simulink model "InterfazOriginalv1Simu2016a"  (R2016a)
settings: Solver=FixedStepAuto  StartTime=10  StopTime=150  FixedStep=0.001  RelTol=1e-3
model workspace (MAT data in the model file):
  g_density = 5
libraries: simulink_extras x9, dspnetwork x7, etargetslib x5, dspfdesign x1
settings Model: Creator=Flight Test Lab  LastModifiedBy=Manolo
settings SolverCC: AutoInsertRateTranBlk=on
settings DataIOCC: SaveFormat=StructureWithTime
settings OptimizationCC: BlockReduction=off  DefaultUnderspecifiedDataType=single  OptimizeBlockIOStorage=off  BufferReuse=off  GlobalBufferReuse=off  ExpressionFolding=off  LocalBlockOutputs=off
settings DebuggingCC: SFUnexpectedBacktrackingDiag=error  SFNoUnconditionalDefaultTransitionDiag=error
settings HardwareCC: ProdWordSize=32  ProdHWDeviceType=Specified
settings RTWCC: Description=Generic Real-Time Target  TargetLang=C++  RTWCompilerOptimization=on
settings CodeAppCC: MaxIdLength=95
settings GRTTargetCC: TargetLangStandard=C++03 (ISO)  GeneratePreprocessorConditionals=Use local settings  MultiInstanceERTCode=on  CodeInterfacePackaging=C++ class
settings ConfigComp: CovMetricSettings=dwe  CovHtmlReporting=off  CovSaveCumulativeToWorkspaceVar=off  CovSaveSingleToWorkspaceVar=off  CovExternalEMLEnable=on

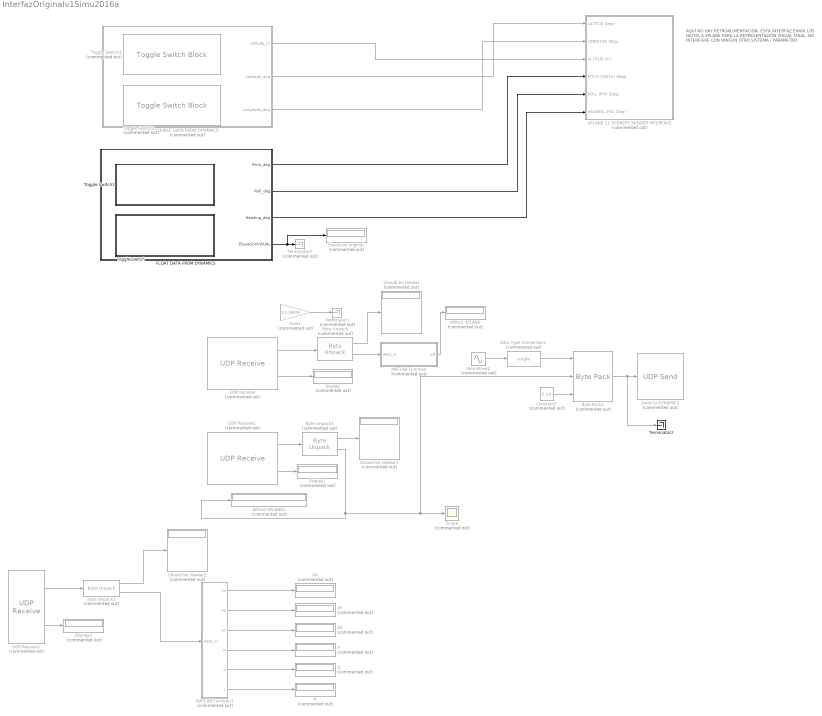
== system InterfazOriginalv1Simu2016a ==
  note: AQUÍ NO HAY RETROALIMENTACIÓN. ESTA INTERFAZ ENVÍA LOS DATOS
      | A XPLANE PARA LA REPRESENTACIÓN VISUAL FINAL, NO INTERFIERE CON
      | NINGUN OTRO SISTEMA / PARÁMETRO
  " DOUBLE DATA FROM DYNAMICS" : Subsystem  Commented=on
  " FLOAT DATA FROM DYNAMICS" : Subsystem
  " XPLANE 11 SCENERY RENDER INTERFACE" : Subsystem  Commented=on
  AX : Display  Commented=on
  AY : Display  Commented=on
  AZ : Display  Commented=on
  Altitud XPLANE : Display  Commented=on
  Altitud XPLANE2 : Display  Commented=on
      settings: Decimation=5
  Byte Pack1 : etargetslib/Byte Pack  Commented=on  datatypes={'single','single','single'}  byteAlign=1
  Byte Unpack : etargetslib/Byte Unpack  Commented=on  dimensions={5,[1,9]}  datatypes={'uint8','single'}  byteAlign=1
  Byte Unpack1 : etargetslib/Byte Unpack  Commented=on  dimensions={5,1}  datatypes={'uint8','single'}  byteAlign=1
  Byte Unpack3 : etargetslib/Byte Unpack  Commented=on  dimensions={5,[9,8]}  datatypes={'uint8','single'}  byteAlign=1
  Constant7 : Constant  Commented=on  Value=5.14  OutDataTypeStr=single
  Data Type Conversion1 : DataTypeConversion  Commented=on  OutDataTypeStr=single
  Display : Display  Commented=on
  Display1 : Display  Commented=on
  Display3 : Display  Commented=on
  Elevacion original : Display  Commented=on
      settings: Decimation=5
  Gain1 : Gain  Commented=on  Gain=1/3.28084
  MATLAB Function : MATLAB Function  Commented=on  TreatAsAtomicUnit=on
  MATLAB Function1 : MATLAB Function  Commented=on  TreatAsAtomicUnit=on
  P : Display  Commented=on
  Q : Display  Commented=on
  R : Display  Commented=on
  Scope : Scope  Commented=on
  Send to DYNAMICS : dspnetwork/UDP Send  Commented=on  remoteURL='1.1.1.1'  remotePort=19750  localURL='0.0.0.0'  localPortSource=Automatically determine  localPort=19750  sampletime=-1  blockPlatform=[]  separateLengthPort=0
  Should be Header : Display  Commented=on
  Should be Header1 : Display  Commented=on
  Should be Header2 : Display  Commented=on
  Sine Wave1 : Sin  Commented=on  Amplitude=90  SampleTime=0
  Terminator1 : Terminator  Commented=on
  Terminator2 : Terminator
  Terminator3 : Terminator  Commented=on
  Toggle Switch : Subsystem  DialogController=hmiCreateDDGDialog  IsWebBlock=on  mask(MWDashboardBlock){webBlockId=9a99a978-ce7c-43f5-ad35-1dbae24a8aa3, webBlockType=toggleswitch, ShowInLibBrowser=on, ShowInitialText=on, HMISrcModelName=InterfazOriginalv1Simu2016a}
      mask prompts: webBlockId "WebBlock Id"; webBlockType "WebBlock Type"; HMISrcModelName "Source Model"
      mask help: Set on/off value to tune parameters or variables.
      mask Help: helpview([docroot '/mapfiles/simulink.map'], 'hmi_switch')
      mask Display:
      | if strcmp(get_param(bdroot(gcb),'BlockDiagramType'),'library')
      |  image([(matlabroot) '/toolbox/simulink/hmi/icons/ToggleSwitch.png'])
      | end
  Toggle Switch1 : Subsystem  DialogController=hmiCreateDDGDialog  IsWebBlock=on  mask(MWDashboardBlock){webBlockId=7adb6560-95fd-42cd-ad0e-2d161efe3a99, webBlockType=toggleswitch, ShowInLibBrowser=on, ShowInitialText=on, HMISrcModelName=InterfazOriginalv1Simu2016a}
      mask prompts: webBlockId "WebBlock Id"; webBlockType "WebBlock Type"; HMISrcModelName "Source Model"
      mask help: Set on/off value to tune parameters or variables.
      mask Help: helpview([docroot '/mapfiles/simulink.map'], 'hmi_switch')
      mask Display:
      | if strcmp(get_param(bdroot(gcb),'BlockDiagramType'),'library')
      |  image([(matlabroot) '/toolbox/simulink/hmi/icons/ToggleSwitch.png'])
      | end
  Toggle Switch2 : ToggleSwitchBlock  Commented=on  WebBlockId=552  LabelPosition=Hide
      settings: Values={{'Replay Archivo', 'Conexión En Tiempo Real'}, [-1 1]}
  Toggle Switch3 : ToggleSwitchBlock  Commented=on  WebBlockId=553  LabelPosition=Hide
      settings: Values={{'No grabar', 'Grabar datos'}, [-1 1]}
  UDP Receive : dspnetwork/UDP Receive  Commented=on  localURL='0.0.0.0'  localPort=49004  remoteURL='127.0.0.1'  remotePort=-1  recvBufferSize=8192  dims=41  signalDatatype=uint8  isVarSize=off  showBlockingTime=off  blockingTime=0  sampletime=inf  blockPlatform=[]
  UDP Receive1 : dspnetwork/UDP Receive  Commented=on  localURL='0.0.0.0'  localPort=49010  remoteURL='127.0.0.1'  remotePort=-1  recvBufferSize=8192  dims=9  signalDatatype=uint8  isVarSize=off  showBlockingTime=off  blockingTime=0  sampletime=inf  blockPlatform=[]
  UDP Receive3 : dspnetwork/UDP Receive  Commented=on  localURL='0.0.0.0'  localPort=49004  remoteURL='127.0.0.1'  remotePort=-1  recvBufferSize=8192  dims=293  signalDatatype=uint8  isVarSize=off  showBlockingTime=off  blockingTime=0  sampletime=inf  blockPlatform=[]
  wires:
  Sine Wave1/1 -> Data Type Conversion1/1
  Constant7/1 -> Byte Pack1/3
  Byte Pack1/1 -> Terminator2/1, Send to DYNAMICS/1
  Data Type Conversion1/1 -> Byte Pack1/1
  UDP Receive/2 -> Display/1
  Byte Unpack/1 -> Should be Header/1
  UDP Receive/1 -> Byte Unpack/1
  Byte Unpack/2 -> MATLAB Function/1(data_in)
  MATLAB Function/1(alt) -> Altitud XPLANE/1
  " DOUBLE DATA FROM DYNAMICS"/2(Latitude_deg) -> " XPLANE 11 SCENERY RENDER INTERFACE"/1(LATITUD (Deg))
  " DOUBLE DATA FROM DYNAMICS"/3(Longitude_deg) -> " XPLANE 11 SCENERY RENDER INTERFACE"/2(LONGITUD (Deg))
  " FLOAT DATA FROM DYNAMICS"/1(Pitch_deg) -> " XPLANE 11 SCENERY RENDER INTERFACE"/4(PITCH (THETA) (Deg))
  " FLOAT DATA FROM DYNAMICS"/2(Roll_deg) -> " XPLANE 11 SCENERY RENDER INTERFACE"/5(ROLL (PHI) (Deg))
  " FLOAT DATA FROM DYNAMICS"/3(Heading_deg) -> " XPLANE 11 SCENERY RENDER INTERFACE"/6(HEADING (PSI) (Deg))
  " DOUBLE DATA FROM DYNAMICS"/1("altitude_m ") -> " XPLANE 11 SCENERY RENDER INTERFACE"/3(ALTITUD (m))
  UDP Receive1/2 -> Display1/1
  UDP Receive1/1 -> Byte Unpack1/1
  Byte Unpack1/1 -> Should be Header1/1
  Byte Unpack1/2 -> Byte Pack1/2, Scope/1, Altitud XPLANE2/1
  " FLOAT DATA FROM DYNAMICS"/4("ElevacionVISUAL ") -> Elevacion original/1, Terminator3/1
  Gain1/1 -> Terminator1/1
  MATLAB Function1/4(p) -> P/1
  MATLAB Function1/6(r) -> R/1
  MATLAB Function1/5(q) -> Q/1
  MATLAB Function1/2(ay) -> AY/1
  MATLAB Function1/3(az) -> AZ/1
  MATLAB Function1/1(ax) -> AX/1
  Byte Unpack3/1 -> Should be Header2/1
  Byte Unpack3/2 -> MATLAB Function1/1(data_in)
  UDP Receive3/1 -> Byte Unpack3/1
  UDP Receive3/2 -> Display3/1

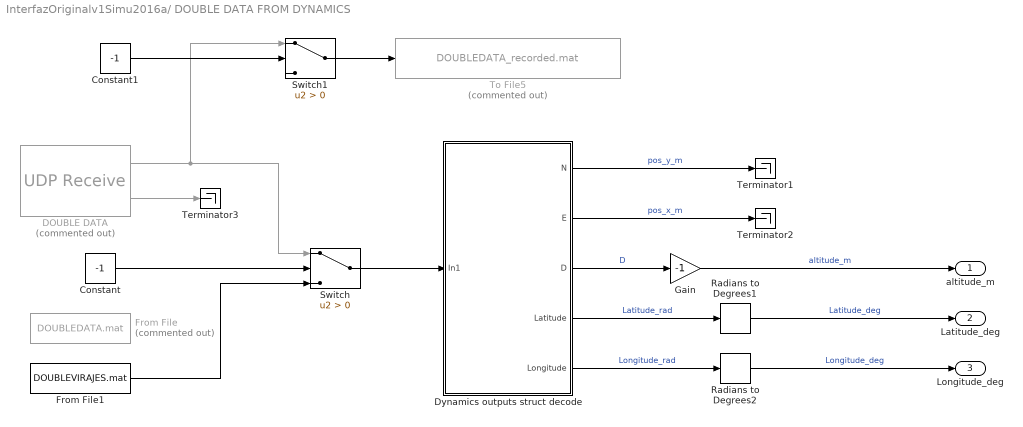
== system InterfazOriginalv1Simu2016a/ DOUBLE DATA FROM DYNAMICS ==
  Constant : Constant  Value=-1
  Constant1 : Constant  Value=-1
  DOUBLE DATA : dspnetwork/UDP Receive  Commented=on  localURL='0.0.0.0'  localPort=19700  remoteURL='0.0.0.0'  remotePort=-1  recvBufferSize=300  dims=5  signalDatatype=double  isVarSize=off  showBlockingTime=on  blockingTime=0  sampletime=0.001  blockPlatform=WINDOWS
  Dynamics outputs struct decode : Subsystem
  From File : FromFile  Commented=on  FileName=DOUBLEDATA.mat
  From File1 : FromFile  FileName=DOUBLEVIRAJES.mat
  Gain : Gain  Gain=-1
  Radians to Degrees1 : simulink_extras/Transformations/Radians to Degrees
  Radians to Degrees2 : simulink_extras/Transformations/Radians to Degrees
  Switch : Switch  Criteria=u2 > Threshold
  Switch1 : Switch  Criteria=u2 > Threshold
  Terminator1 : Terminator
  Terminator2 : Terminator
  Terminator3 : Terminator
  To File5 : ToFile  Commented=on  Filename=DOUBLEDATA_recorded.mat  MatrixName=DOUBLEDATA_recorded  SaveFormat=Timeseries  SampleTime=0.001
      settings: Decimation=16
  "altitude_m " : Outport
  Latitude_deg : Outport  Port=2
  Longitude_deg : Outport  Port=3
  wires:
  Dynamics outputs struct decode/3(D) -> Gain/1  "D"
  Dynamics outputs struct decode/1(N) -> Terminator1/1  "pos_y_m"
  Dynamics outputs struct decode/4("Latitude ") -> Radians to Degrees1/1  "Latitude_rad"
  Dynamics outputs struct decode/5(Longitude) -> Radians to Degrees2/1  "Longitude_rad"
  Dynamics outputs struct decode/2(E) -> Terminator2/1  "pos_x_m"
  Gain/1 -> "altitude_m "/1  "altitude_m"
  Radians to Degrees1/1 -> Latitude_deg/1  "Latitude_deg"
  Radians to Degrees2/1 -> Longitude_deg/1  "Longitude_deg"
  DOUBLE DATA/2 -> Terminator3/1
  Constant/1 -> Switch/2
  DOUBLE DATA/1 -> Switch1/1, Switch/1
  Switch/1 -> Dynamics outputs struct decode/1(In1)
  Switch1/1 -> To File5/1
  Constant1/1 -> Switch1/2
  From File1/1 -> Switch/3

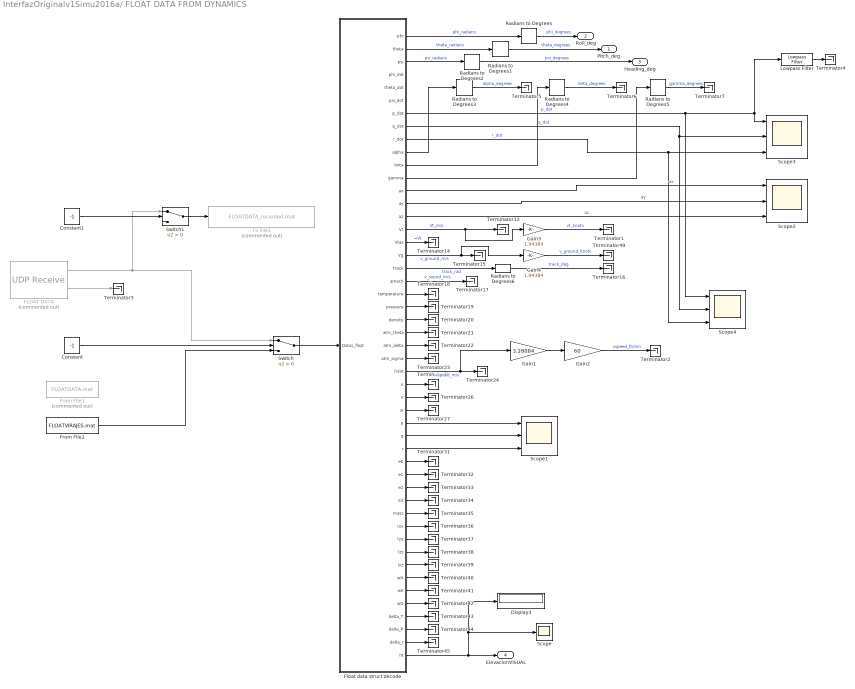
== system InterfazOriginalv1Simu2016a/ FLOAT DATA FROM DYNAMICS ==
  Constant : Constant  Value=-1
  Constant1 : Constant  Value=-1
  Display3 : Display
  FLOAT DATA : dspnetwork/UDP Receive  Commented=on  localURL='0.0.0.0'  localPort=19600  remoteURL='0.0.0.0'  remotePort=-1  recvBufferSize=1000  dims=49  signalDatatype=single  isVarSize=off  showBlockingTime=on  blockingTime=0  sampletime=0.001  blockPlatform=WINDOWS
  Float data struct decode : Subsystem
  From File1 : FromFile  Commented=on  FileName=FLOATDATA.mat  SampleTime=0.001
  From File2 : FromFile  FileName=FLOATVIRAJES.mat  SampleTime=0.001
  Gain1 : Gain  Gain=3.28084
  Gain2 : Gain  Gain=60
  Gain3 : Gain  Gain=1.94384
  Gain4 : Gain  Gain=1.94384
  Lowpass Filter : dspfdesign/Lowpass Filter  FilterType=IIR  DesignForMinimumOrder=on  FilterOrder=50  PassbandFrequency=1  StopbandFrequency=35  PassbandRipple=0.1  StopbandAttenuation=40  InheritSampleRate=on  SampleRate=44100  SimulateUsing=Interpreted execution  roundingMode=Floor  coeffsDataTypeStr=fixdt(1,16)
  Radians to Degrees{,1..6} (7 alike) : simulink_extras/Transformations/Radians to Degrees
  Scope : Scope
  Scope{1..4} (4 alike) : Scope  NumInputPorts=3
  Switch : Switch  Criteria=u2 > Threshold
  Switch1 : Switch  Criteria=u2 > Threshold
  Terminator{1..7,13..27,31..45,49} (38 alike) : Terminator
  To File1 : ToFile  Commented=on  Filename=FLOATDATA_recorded.mat  MatrixName=FOATDATA_recorded  SaveFormat=Timeseries  SampleTime=0.001
      settings: Decimation=6
  Pitch_deg : Outport
  Roll_deg : Outport  Port=2
  Heading_deg : Outport  Port=3
  "ElevacionVISUAL " : Outport  Port=4
  wires:
  Float data struct decode/1(phi) -> Radians to Degrees/1  "phi_radians"
  Float data struct decode/2(theta) -> Radians to Degrees1/1  "theta_radians"
  Float data struct decode/3("psi ") -> Radians to Degrees2/1  "psi_radians"
  Float data struct decode/10(alpha) -> Radians to Degrees3/1
  Float data struct decode/11(beta) -> Radians to Degrees4/1
  Float data struct decode/12(gamma) -> Radians to Degrees5/1
  Radians to Degrees/1 -> Roll_deg/1  "phi_degrees"
  Radians to Degrees2/1 -> Heading_deg/1  "psi_degrees"
  Radians to Degrees1/1 -> Pitch_deg/1  "theta_degrees"
  Radians to Degrees3/1 -> Terminator5/1  "alpha_degrees"
  Radians to Degrees4/1 -> Terminator6/1  "beta_degrees"
  Radians to Degrees5/1 -> Terminator7/1  "gamma_degrees"
  Float data struct decode/17(Vtas) -> Terminator14/1  "=Vt"
  Float data struct decode/18(Vg) -> Gain4/1, Terminator15/1  "v_ground_m/s"
  Float data struct decode/19(track) -> Radians to Degrees6/1  "track_rad"
  Float data struct decode/20(amach) -> Terminator17/1  "v_sound_m/s"
  Float data struct decode/21(temperature) -> Terminator18/1
  Float data struct decode/22(pressure) -> Terminator19/1
  Float data struct decode/23(density) -> Terminator20/1
  Float data struct decode/24(atm_theta) -> Terminator21/1
  Float data struct decode/25(atm_delta) -> Terminator22/1
  Float data struct decode/26(atm_sigma) -> Terminator23/1
  Float data struct decode/28(u) -> Terminator25/1
  Float data struct decode/29(v) -> Terminator26/1
  Float data struct decode/30(w) -> Terminator27/1
  Float data struct decode/31(p) -> Scope1/1
  Float data struct decode/32(q) -> Scope1/2
  Float data struct decode/33(r) -> Scope1/3
  Float data struct decode/34(e0) -> Terminator31/1
  Float data struct decode/35(e1) -> Terminator32/1
  Float data struct decode/36(e2) -> Terminator33/1
  Float data struct decode/37(e3) -> Terminator34/1
  Float data struct decode/38(mass) -> Terminator35/1
  Float data struct decode/39(Ixx) -> Terminator36/1
  Float data struct decode/40(Iyy) -> Terminator37/1
  Float data struct decode/41(Izz) -> Terminator38/1
  Float data struct decode/42(Ixz) -> Terminator39/1
  Float data struct decode/43(wN) -> Terminator40/1
  Float data struct decode/44(wE) -> Terminator41/1
  Float data struct decode/45(wD) -> Terminator42/1
  Float data struct decode/46(delta_T) -> Terminator43/1
  Float data struct decode/47(delta_P) -> Terminator44/1
  Float data struct decode/48(delta_r) -> Terminator45/1
  Float data struct decode/49(ht) -> Scope/1, Display3/1, "ElevacionVISUAL "/1
  Float data struct decode/27(hdot) -> Gain1/1, Terminator24/1  "vspeed_m/s"
  Gain1/1 -> Gain2/1
  Gain2/1 -> Terminator2/1  "vspeed_ft/min"
  Float data struct decode/16(Vt) -> Gain3/1, Terminator13/1  "Vt_m/s"
  Gain3/1 -> Terminator1/1  "vt_knots"
  Gain4/1 -> Terminator49/1  "v_ground_knots"
  Radians to Degrees6/1 -> Terminator16/1  "track_deg"
  FLOAT DATA/2 -> Terminator3/1
  Switch/1 -> Float data struct decode/1(Datos_float)
  FLOAT DATA/1 -> Switch1/1, Switch/1
  Constant/1 -> Switch/2
  Switch1/1 -> To File1/1
  Constant1/1 -> Switch1/2
  Float data struct decode/7(p_dot) -> Scope4/1, Lowpass Filter/1, Scope3/1  "p_dot"
  Lowpass Filter/1 -> Terminator4/1
  Float data struct decode/8(q_dot) -> Scope4/2, Scope3/2  "q_dot"
  Float data struct decode/9(r_dot) -> Scope4/3, Scope3/3  "r_dot"
  Float data struct decode/13(ax) -> Scope2/1  "ax"
  Float data struct decode/14(ay) -> Scope2/2  "ay"
  Float data struct decode/15(az) -> Scope2/3  "az"
  From File2/1 -> Switch/3

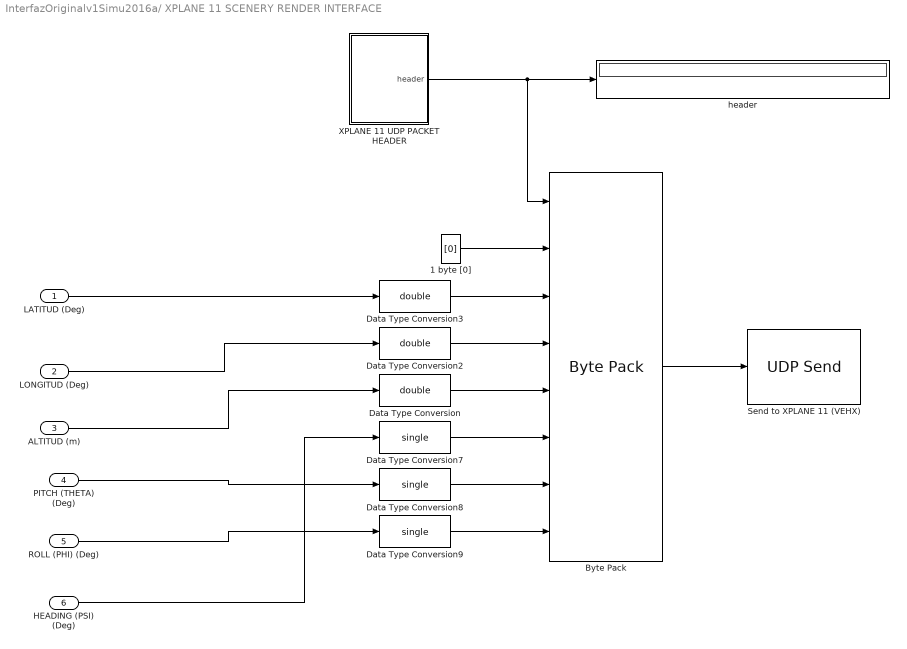
== system InterfazOriginalv1Simu2016a/ XPLANE 11 SCENERY RENDER INTERFACE ==
  LATITUD (Deg) : Inport
  LONGITUD (Deg) : Inport  Port=2
  ALTITUD (m) : Inport  Port=3
  PITCH (THETA) (Deg) : Inport  Port=4
  ROLL (PHI) (Deg) : Inport  Port=5
  HEADING (PSI) (Deg) : Inport  Port=6
  1 byte [0] : Constant  Value=[0]  OutDataTypeStr=single
  Byte Pack : etargetslib/Byte Pack  datatypes={'uint8','single','double','double','double','single','single','single'}  byteAlign=1
  Data Type Conversion : DataTypeConversion  OutDataTypeStr=double
  Data Type Conversion2 : DataTypeConversion  OutDataTypeStr=double
  Data Type Conversion3 : DataTypeConversion  OutDataTypeStr=double
  Data Type Conversion7 : DataTypeConversion  OutDataTypeStr=single
  Data Type Conversion8 : DataTypeConversion  OutDataTypeStr=single
  Data Type Conversion9 : DataTypeConversion  OutDataTypeStr=single
  Send to XPLANE 11 (VEHX) : dspnetwork/UDP Send  remoteURL='127.0.0.1'  remotePort=49000  localURL='0.0.0.0'  localPortSource=Automatically determine  localPort=-1  sampletime=-1  blockPlatform=[]  separateLengthPort=0
  XPLANE 11 UDP PACKET HEADER : MATLAB Function  TreatAsAtomicUnit=on
  header : Display
  wires:
  XPLANE 11 UDP PACKET HEADER/1(header) -> Byte Pack/1, header/1
  Data Type Conversion8/1 -> Byte Pack/7
  1 byte [0]/1 -> Byte Pack/2
  Data Type Conversion9/1 -> Byte Pack/8
  Data Type Conversion/1 -> Byte Pack/5
  Data Type Conversion2/1 -> Byte Pack/4
  Data Type Conversion3/1 -> Byte Pack/3
  Data Type Conversion7/1 -> Byte Pack/6
  HEADING (PSI) (Deg)/1 -> Data Type Conversion7/1
  Byte Pack/1 -> Send to XPLANE 11 (VEHX)/1
  ALTITUD (m)/1 -> Data Type Conversion/1
  LONGITUD (Deg)/1 -> Data Type Conversion2/1
  ROLL (PHI) (Deg)/1 -> Data Type Conversion9/1
  LATITUD (Deg)/1 -> Data Type Conversion3/1
  PITCH (THETA) (Deg)/1 -> Data Type Conversion8/1

== system InterfazOriginalv1Simu2016a/Toggle Switch ==

== system InterfazOriginalv1Simu2016a/Toggle Switch1 ==

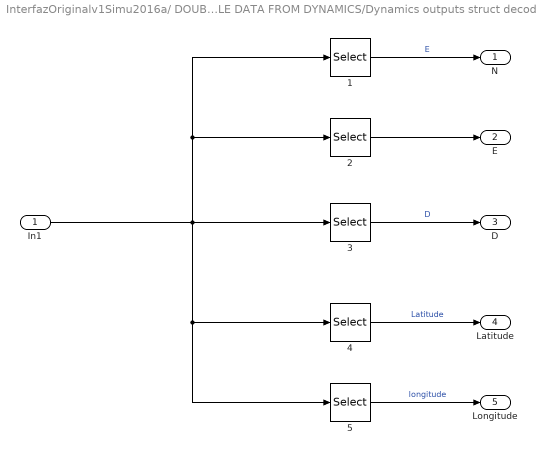
== system InterfazOriginalv1Simu2016a/ DOUBLE DATA FROM DYNAMICS/Dynamics outputs struct decode ==
  In1 : Inport
  1 : Selector  InputPortWidth=5  IndexOptions=Index vector (dialog)  Indices=[1]  OutputSizes=1
  2 : Selector  InputPortWidth=5  IndexOptions=Index vector (dialog)  Indices=[2]  OutputSizes=1
  3 : Selector  InputPortWidth=5  IndexOptions=Index vector (dialog)  Indices=[3]  OutputSizes=1
  4 : Selector  InputPortWidth=5  IndexOptions=Index vector (dialog)  Indices=[4]  OutputSizes=1
  5 : Selector  InputPortWidth=5  IndexOptions=Index vector (dialog)  Indices=[5]  OutputSizes=1
  N : Outport
  E : Outport  Port=2
  D : Outport  Port=3
  "Latitude " : Outport  Port=4
  Longitude : Outport  Port=5
  wires:
  1/1 -> N/1  "E"
  2/1 -> E/1
  3/1 -> D/1  "D"
  In1/1 -> 1/1, 2/1, 5/1, 4/1, 3/1
  4/1 -> "Latitude "/1  "Latitude"
  5/1 -> Longitude/1  "longitude"

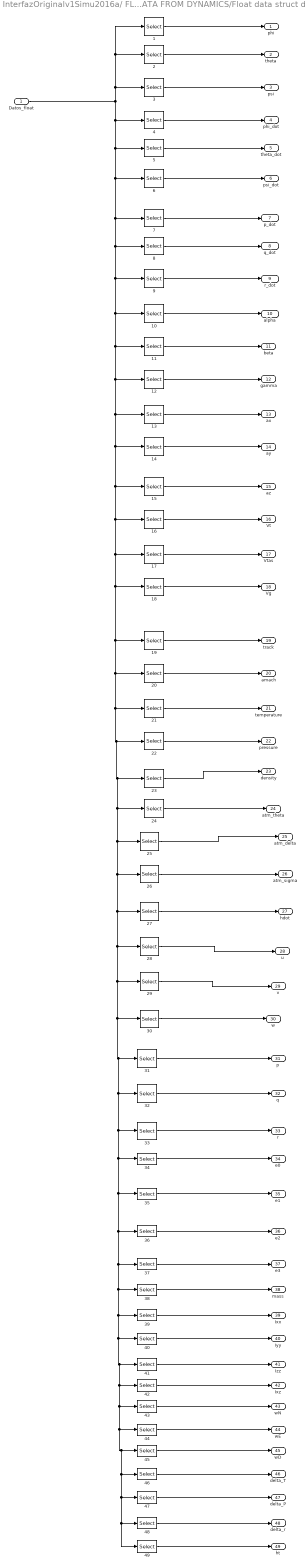
== system InterfazOriginalv1Simu2016a/ FLOAT DATA FROM DYNAMICS/Float data struct decode ==
  Datos_float : Inport
  1 : Selector  InputPortWidth=49  IndexOptions=Index vector (dialog)  Indices=[1]  OutputSizes=1
  10 : Selector  InputPortWidth=49  IndexOptions=Index vector (dialog)  Indices=[10]  OutputSizes=1
  11 : Selector  InputPortWidth=49  IndexOptions=Index vector (dialog)  Indices=[11]  OutputSizes=1
  12 : Selector  InputPortWidth=49  IndexOptions=Index vector (dialog)  Indices=[12]  OutputSizes=1
  13 : Selector  InputPortWidth=49  IndexOptions=Index vector (dialog)  Indices=[13]  OutputSizes=1
  14 : Selector  InputPortWidth=49  IndexOptions=Index vector (dialog)  Indices=[14]  OutputSizes=1
  15 : Selector  InputPortWidth=49  IndexOptions=Index vector (dialog)  Indices=[15]  OutputSizes=1
  16 : Selector  InputPortWidth=49  IndexOptions=Index vector (dialog)  Indices=[16]  OutputSizes=1
  17 : Selector  InputPortWidth=49  IndexOptions=Index vector (dialog)  Indices=[17]  OutputSizes=1
  18 : Selector  InputPortWidth=49  IndexOptions=Index vector (dialog)  Indices=[18]  OutputSizes=1
  19 : Selector  InputPortWidth=49  IndexOptions=Index vector (dialog)  Indices=[19]  OutputSizes=1
  2 : Selector  InputPortWidth=49  IndexOptions=Index vector (dialog)  Indices=[2]  OutputSizes=1
  20 : Selector  InputPortWidth=49  IndexOptions=Index vector (dialog)  Indices=[20]  OutputSizes=1
  21 : Selector  InputPortWidth=49  IndexOptions=Index vector (dialog)  Indices=[21]  OutputSizes=1
  22 : Selector  InputPortWidth=49  IndexOptions=Index vector (dialog)  Indices=[22]  OutputSizes=1
  23 : Selector  InputPortWidth=49  IndexOptions=Index vector (dialog)  Indices=[23]  OutputSizes=1
  24 : Selector  InputPortWidth=49  IndexOptions=Index vector (dialog)  Indices=[24]  OutputSizes=1
  25 : Selector  InputPortWidth=49  IndexOptions=Index vector (dialog)  Indices=[25]  OutputSizes=1
  26 : Selector  InputPortWidth=49  IndexOptions=Index vector (dialog)  Indices=[26]  OutputSizes=1
  27 : Selector  InputPortWidth=49  IndexOptions=Index vector (dialog)  Indices=[27]  OutputSizes=1
  28 : Selector  InputPortWidth=49  IndexOptions=Index vector (dialog)  Indices=[28]  OutputSizes=1
  29 : Selector  InputPortWidth=49  IndexOptions=Index vector (dialog)  Indices=[29]  OutputSizes=1
  3 : Selector  InputPortWidth=49  IndexOptions=Index vector (dialog)  Indices=[3]  OutputSizes=1
  30 : Selector  InputPortWidth=49  IndexOptions=Index vector (dialog)  Indices=[30]  OutputSizes=1
  31 : Selector  InputPortWidth=49  IndexOptions=Index vector (dialog)  Indices=[31]  OutputSizes=1
  32 : Selector  InputPortWidth=49  IndexOptions=Index vector (dialog)  Indices=[32]  OutputSizes=1
  33 : Selector  InputPortWidth=49  IndexOptions=Index vector (dialog)  Indices=[33]  OutputSizes=1
  34 : Selector  InputPortWidth=49  IndexOptions=Index vector (dialog)  Indices=[34]  OutputSizes=1
  35 : Selector  InputPortWidth=49  IndexOptions=Index vector (dialog)  Indices=[35]  OutputSizes=1
  36 : Selector  InputPortWidth=49  IndexOptions=Index vector (dialog)  Indices=[36]  OutputSizes=1
  37 : Selector  InputPortWidth=49  IndexOptions=Index vector (dialog)  Indices=[37]  OutputSizes=1
  38 : Selector  InputPortWidth=49  IndexOptions=Index vector (dialog)  Indices=[38]  OutputSizes=1
  39 : Selector  InputPortWidth=49  IndexOptions=Index vector (dialog)  Indices=[39]  OutputSizes=1
  4 : Selector  InputPortWidth=49  IndexOptions=Index vector (dialog)  Indices=[4]  OutputSizes=1
  40 : Selector  InputPortWidth=49  IndexOptions=Index vector (dialog)  Indices=[40]  OutputSizes=1
  41 : Selector  InputPortWidth=49  IndexOptions=Index vector (dialog)  Indices=[41]  OutputSizes=1
  42 : Selector  InputPortWidth=49  IndexOptions=Index vector (dialog)  Indices=[42]  OutputSizes=1
  43 : Selector  InputPortWidth=49  IndexOptions=Index vector (dialog)  Indices=[43]  OutputSizes=1
  44 : Selector  InputPortWidth=49  IndexOptions=Index vector (dialog)  Indices=[44]  OutputSizes=1
  45 : Selector  InputPortWidth=49  IndexOptions=Index vector (dialog)  Indices=[45]  OutputSizes=1
  46 : Selector  InputPortWidth=49  IndexOptions=Index vector (dialog)  Indices=[46]  OutputSizes=1
  47 : Selector  InputPortWidth=49  IndexOptions=Index vector (dialog)  Indices=[47]  OutputSizes=1
  48 : Selector  InputPortWidth=49  IndexOptions=Index vector (dialog)  Indices=[48]  OutputSizes=1
  49 : Selector  InputPortWidth=49  IndexOptions=Index vector (dialog)  Indices=[49]  OutputSizes=1
  5 : Selector  InputPortWidth=49  IndexOptions=Index vector (dialog)  Indices=[5]  OutputSizes=1
  6 : Selector  InputPortWidth=49  IndexOptions=Index vector (dialog)  Indices=[6]  OutputSizes=1
  7 : Selector  InputPortWidth=49  IndexOptions=Index vector (dialog)  Indices=[7]  OutputSizes=1
  8 : Selector  InputPortWidth=49  IndexOptions=Index vector (dialog)  Indices=[8]  OutputSizes=1
  9 : Selector  InputPortWidth=49  IndexOptions=Index vector (dialog)  Indices=[9]  OutputSizes=1
  phi : Outport
  theta : Outport  Port=2
  "psi " : Outport  Port=3
  phi_dot : Outport  Port=4
  theta_dot : Outport  Port=5
  psi_dot : Outport  Port=6
  p_dot : Outport  Port=7
  q_dot : Outport  Port=8
  r_dot : Outport  Port=9
  alpha : Outport  Port=10
  beta : Outport  Port=11
  gamma : Outport  Port=12
  ax : Outport  Port=13
  ay : Outport  Port=14
  az : Outport  Port=15
  Vt : Outport  Port=16
  Vtas : Outport  Port=17
  Vg : Outport  Port=18
  track : Outport  Port=19
  amach : Outport  Port=20
  temperature : Outport  Port=21
  pressure : Outport  Port=22
  density : Outport  Port=23
  atm_theta : Outport  Port=24
  atm_delta : Outport  Port=25
  atm_sigma : Outport  Port=26
  hdot : Outport  Port=27
  u : Outport  Port=28
  v : Outport  Port=29
  w : Outport  Port=30
  p : Outport  Port=31
  q : Outport  Port=32
  r : Outport  Port=33
  e0 : Outport  Port=34
  e1 : Outport  Port=35
  e2 : Outport  Port=36
  e3 : Outport  Port=37
  mass : Outport  Port=38
  Ixx : Outport  Port=39
  Iyy : Outport  Port=40
  Izz : Outport  Port=41
  Ixz : Outport  Port=42
  wN : Outport  Port=43
  wE : Outport  Port=44
  wD : Outport  Port=45
  delta_T : Outport  Port=46
  delta_P : Outport  Port=47
  delta_r : Outport  Port=48
  ht : Outport  Port=49
  wires:
  4/1 -> phi_dot/1
  1/1 -> phi/1
  2/1 -> theta/1
  3/1 -> "psi "/1
  5/1 -> theta_dot/1
  6/1 -> psi_dot/1
  7/1 -> p_dot/1
  8/1 -> q_dot/1
  9/1 -> r_dot/1
  10/1 -> alpha/1
  11/1 -> beta/1
  12/1 -> gamma/1
  13/1 -> ax/1
  14/1 -> ay/1
  18/1 -> Vg/1
  17/1 -> Vtas/1
  15/1 -> az/1
  16/1 -> Vt/1
  22/1 -> pressure/1
  19/1 -> track/1
  21/1 -> temperature/1
  20/1 -> amach/1
  23/1 -> density/1
  24/1 -> atm_theta/1
  25/1 -> atm_delta/1
  26/1 -> atm_sigma/1
  31/1 -> p/1
  32/1 -> q/1
  30/1 -> w/1
  29/1 -> v/1
  28/1 -> u/1
  27/1 -> hdot/1
  33/1 -> r/1
  Datos_float/1 -> 6/1, 48/1, 49/1, 47/1, 46/1, 45/1, 44/1, 43/1, 42/1, 41/1, 40/1, 39/1, 38/1, 37/1, 36/1, 35/1, 34/1, 33/1, 32/1, 31/1, 30/1, 29/1, 28/1, 27/1, 26/1, 25/1, 24/1, 23/1, 22/1, 21/1, 20/1, 19/1, 18/1, 17/1, 16/1, 15/1, 14/1, 13/1, 12/1, 11/1, 10/1, 9/1, 8/1, 7/1, 5/1, 4/1, 3/1, 2/1, 1/1
  34/1 -> e0/1
  35/1 -> e1/1
  36/1 -> e2/1
  37/1 -> e3/1
  39/1 -> Ixx/1
  38/1 -> mass/1
  40/1 -> Iyy/1
  41/1 -> Izz/1
  42/1 -> Ixz/1
  43/1 -> wN/1
  44/1 -> wE/1
  45/1 -> wD/1
  46/1 -> delta_T/1
  47/1 -> delta_P/1
  48/1 -> delta_r/1
  49/1 -> ht/1

== matlab function InterfazOriginalv1Simu2016a/ XPLANE 11 SCENERY RENDER INTERFACE/XPLANE 11 UDP PACKET HEADER ==
  data: header output uint8
function header  = fcn 
header =[uint8(86) uint8(69) uint8(72) uint8(88) uint8(48)];

 %Surface_header = typecast(uint8([uint8(8) uint8(0) uint8(0) uint8(0)]),'single')
%surfaces_control_cmd = [0 dat_lat dat_lon dat_ele veh_psi_true veh_the veh_phi];
%Throttle_header = typecast(uint8([uint8(25) uint8(0) uint8(0) uint8(0)]),'single');
%throttle_cmd = [3.503246160812043e-44 throttle No_Comand No_Comand No_Comand No_Comand No_Comand No_Comand No_Comand];
end

== matlab function InterfazOriginalv1Simu2016a/MATLAB Function ==
  data: data_in input; alt output
function alt  = decoder(data_in)
 alt = data_in(1,4);
 alt = data_in(1,4);
 alt = data_in(1,4);
 alt = data_in(1,4);
 alt = data_in(1,4);
 

end

== matlab function InterfazOriginalv1Simu2016a/MATLAB Function1 ==
  data: data_in input; ax output; ay output; az output; p output; q output; r output
function [ax, ay, az,...
    p, q, r] = decoder(data_in)

  p= data_in(5,1); 
  q= data_in(6,1);
  r= data_in(7,1);
 ax= data_in(2,1);
 ay= data_in(3,1);
 az= data_in(4,1);

end
